simulink model "temp_control"  (Simulink 8.7)
settings: Solver=ode45  StartTime=0.0  StopTime=20000  RelTol=1e-4
settings Model: Creator=EliteBook 8470p  LastModifiedBy=EliteBook 8470p
settings DataIOCC: SignalLoggingSaveFormat=ModelDataLogs
settings OptimizationCC: BlockReduction=off  BooleanDataType=off
settings DebuggingCC: SaveWithParameterizedLinksMsg=none  SignalResolutionControl=TryResolveAllWithWarning  MultiTaskDSMMsg=warning  MultiTaskCondExecSysMsg=none
settings HardwareCC: ProdBitPerPointer=64  ProdLargestAtomicFloat=Float  ProdIntDivRoundTo=Zero  ProdEndianess=LittleEndian  ProdWordSize=64  ProdHWDeviceType=Intel->x86-64 (Windows64)  TargetUnknown=on
settings GRTTargetCC: GeneratePreprocessorConditionals=Use local settings  CombineOutputUpdateFcns=off  GRTInterface=on

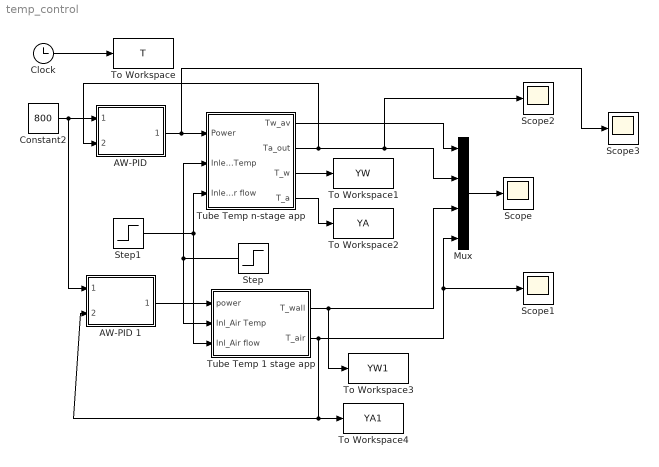
== system temp_control ==
  "AW-PID " : Subsystem  mask(Anti-windup PID){}
      mask help: Discrete PID with Anti-windup and with lowpass filter
      mask init:
      | kp=@1(1);ki=@1(2);kd=@1(3);SAM=@2;TF=@3;DT=@4;umax=@5(1);umin=@5(2);
      mask Display: disp('AW-PID+filter')
  AW-PID 1 : Subsystem  mask(Anti-windup PID){}
      mask help: Discrete PID with Anti-windup and with lowpass filter
      mask init:
      | kp=@1(1);ki=@1(2);kd=@1(3);SAM=@2;TF=@3;DT=@4;umax=@5(1);umin=@5(2);
      mask Display: disp('AW-PID+filter')
  Clock : Clock
  Constant2 : Constant  Value=800
  Mux : Mux
  Scope{,1..3} (4 alike) : Scope
  Step : Step  Time=10000  Before=25  After=500  SampleTime=0
  Step1 : Step  Time=5000  Before=1  After=10  SampleTime=0
  To Workspace : ToWorkspace  VariableName=T  SampleTime=1
  To Workspace1 : ToWorkspace  VariableName=YW  SampleTime=1
  To Workspace2 : ToWorkspace  VariableName=YA  SampleTime=1
  To Workspace3 : ToWorkspace  VariableName=YW1  SampleTime=1
  To Workspace4 : ToWorkspace  VariableName=YA1  SampleTime=1
  Tube Temp 1 stage app : Subsystem  mask{L=1, ra=.1, T_0=25, T_a0=25, T_amb=25}
      mask prompts: L "Tube length"; ra "Tube inner radius"; T_0 "Initial Tube temp"; T_a0 "Initial Air Temp"; T_amb "Ambient Temp"
      mask init:
      | cp=1078;cpa=1134;rhoa=0.5;k=2;hs=5;ha=30;
      | rhos=2500;d=.01;vt=pi*L*((ra+d)*(ra+d)-ra*ra);m=vt*rhos;
      | As=2*pi*(ra+.1)*L;V=pi*ra*ra*L;Aa=2*pi*ra*L;
      | A_d=pi*((ra+d)*(ra+d)-ra*ra);
  Tube Temp n-stage app : Subsystem  mask{L=1, n=100, ra=.1, T_01=25, T_a01=25, T_amb=25}
      mask prompts: L "Tube Length"; n "Number of sections"; ra "Tube inner radius"; T_01 "Initial tube temp"; T_a01 "Initial air temp"; T_amb "Ambient Temp"
      mask init:
      | cp=1078;cpa=1134;rhoa=0.5;hs=5;ha=30;rhos=2500;k=2;
      | d=.01;vt=pi*L*((ra+d)*(ra+d)-ra*ra);m=vt*rhos;
      | As=2*pi*(ra+.1)*L;V=pi*ra*ra*L;Aa=2*pi*ra*L;
      | A_d=pi*((ra+d)*(ra+d)-ra*ra);A_rat=1;Li=L/n;
      | T_0=T_01*ones(n,1);T_a0=T_a01*ones(n,1);
  wires:
  Mux/1 -> Scope/1
  Tube Temp 1 stage app/1(T_wall) -> Mux/3, To Workspace3/1
  Tube Temp 1 stage app/2(T_air) -> Mux/4, Scope1/1, To Workspace4/1, AW-PID 1/2(System Output)
  Tube Temp n-stage app/1(Tw_av) -> Mux/1
  Tube Temp n-stage app/2(Ta_out) -> Scope2/1, Mux/2, "AW-PID "/2(System Output)
  Clock/1 -> To Workspace/1
  Tube Temp n-stage app/3(T_w) -> To Workspace1/1
  Tube Temp n-stage app/4(T_a) -> To Workspace2/1
  Step/1 -> Tube Temp 1 stage app/2(Inl_Air Temp), Tube Temp n-stage app/2(Inlet Air Temp)
  Constant2/1 -> "AW-PID "/1(Set point), AW-PID 1/1(Set point)
  Step1/1 -> Tube Temp n-stage app/3(Inlet Air flow), Tube Temp 1 stage app/3(Inl_Air flow)
  AW-PID 1/1(Input to system) -> Tube Temp 1 stage app/1(power)
  "AW-PID "/1(Input to system) -> Scope3/1, Tube Temp n-stage app/1(Power)

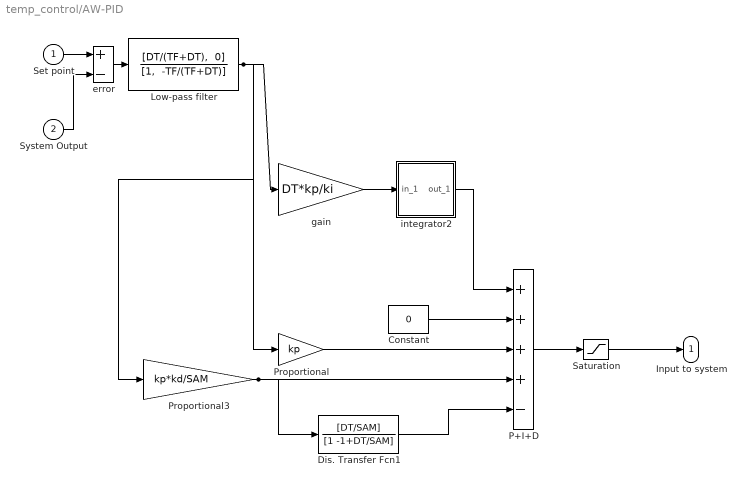
== system temp_control/AW-PID  ==
  Set point : Inport
  System Output : Inport  Port=2
  Constant : Constant  Value=0
  Dis. Transfer Fcn1 : DiscreteTransferFcn  Numerator=[DT/SAM]  Denominator=[1 -1+DT/SAM]  SampleTime=DT
  Low-pass filter : DiscreteTransferFcn  Numerator="[DT/(TF+DT),  0]"  Denominator="[1,  -TF/(TF+DT)]"  SampleTime=DT
  P+I+D : Sum  Inputs=++++-  SaturateOnIntegerOverflow=on  InputSameDT=on  OutDataTypeStr=Inherit: Same as first input
  Proportional : Gain  Gain=kp  SaturateOnIntegerOverflow=on  OutDataTypeStr=Inherit: Same as input  ParamDataTypeStr=Inherit: Same as input
  Proportional3 : Gain  Gain=kp*kd/SAM  SaturateOnIntegerOverflow=on  OutDataTypeStr=Inherit: Same as input  ParamDataTypeStr=Inherit: Same as input
  Saturation : Saturate  UpperLimit=umax  LowerLimit=umin
  error : Sum  Inputs=+-  SaturateOnIntegerOverflow=on  InputSameDT=on  OutDataTypeStr=Inherit: Same as first input
  gain : Gain  Gain=DT*kp/ki  SaturateOnIntegerOverflow=on  OutDataTypeStr=Inherit: Same as input  ParamDataTypeStr=Inherit: Same as input
  integrator2 : Subsystem  mask(Anti windup intgrator){umax=umax, umin=umin, DT=DT}
      mask prompts: DT "sampling time"
      mask help: Integral with anti-windup
      mask Display: disp('DT-I-AW')
  Input to system : Outport  InitialOutput=0
  wires:
  integrator2/1(out_1) -> P+I+D/1
  error/1 -> Low-pass filter/1
  Set point/1 -> error/1
  System Output/1 -> error/2
  Proportional3/1 -> Dis. Transfer Fcn1/1, P+I+D/4
  Low-pass filter/1 -> Proportional/1, Proportional3/1, gain/1
  Dis. Transfer Fcn1/1 -> P+I+D/5
  Proportional/1 -> P+I+D/3
  gain/1 -> integrator2/1(in_1)
  P+I+D/1 -> Saturation/1
  Saturation/1 -> Input to system/1
  Constant/1 -> P+I+D/2

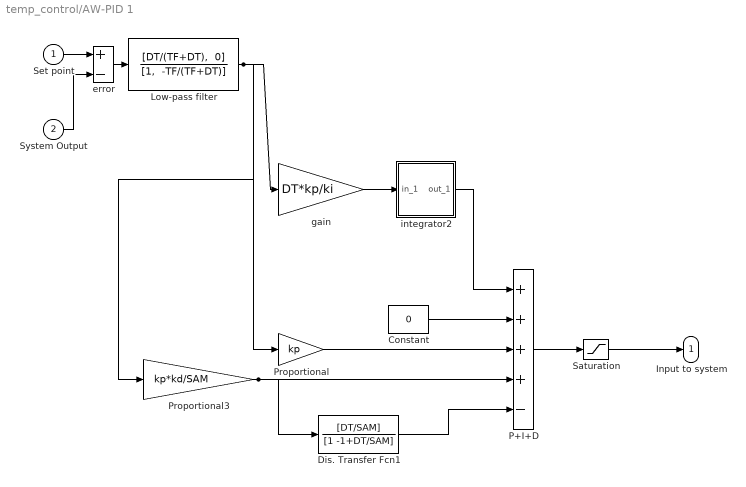
== system temp_control/AW-PID 1 ==
  Set point : Inport
  System Output : Inport  Port=2
  Constant : Constant  Value=0
  Dis. Transfer Fcn1 : DiscreteTransferFcn  Numerator=[DT/SAM]  Denominator=[1 -1+DT/SAM]  SampleTime=DT
  Low-pass filter : DiscreteTransferFcn  Numerator="[DT/(TF+DT),  0]"  Denominator="[1,  -TF/(TF+DT)]"  SampleTime=DT
  P+I+D : Sum  Inputs=++++-  SaturateOnIntegerOverflow=on  InputSameDT=on  OutDataTypeStr=Inherit: Same as first input
  Proportional : Gain  Gain=kp  SaturateOnIntegerOverflow=on  OutDataTypeStr=Inherit: Same as input  ParamDataTypeStr=Inherit: Same as input
  Proportional3 : Gain  Gain=kp*kd/SAM  SaturateOnIntegerOverflow=on  OutDataTypeStr=Inherit: Same as input  ParamDataTypeStr=Inherit: Same as input
  Saturation : Saturate  UpperLimit=umax  LowerLimit=umin
  error : Sum  Inputs=+-  SaturateOnIntegerOverflow=on  InputSameDT=on  OutDataTypeStr=Inherit: Same as first input
  gain : Gain  Gain=DT*kp/ki  SaturateOnIntegerOverflow=on  OutDataTypeStr=Inherit: Same as input  ParamDataTypeStr=Inherit: Same as input
  integrator2 : Subsystem  mask(Anti windup intgrator){umax=umax, umin=umin, DT=DT}
      mask prompts: DT "sampling time"
      mask help: Integral with anti-windup
      mask Display: disp('DT-I-AW')
  Input to system : Outport  InitialOutput=0
  wires:
  Constant/1 -> P+I+D/2
  Saturation/1 -> Input to system/1
  P+I+D/1 -> Saturation/1
  gain/1 -> integrator2/1(in_1)
  Proportional/1 -> P+I+D/3
  Dis. Transfer Fcn1/1 -> P+I+D/5
  Low-pass filter/1 -> gain/1, Proportional3/1, Proportional/1
  Proportional3/1 -> P+I+D/4, Dis. Transfer Fcn1/1
  System Output/1 -> error/2
  Set point/1 -> error/1
  error/1 -> Low-pass filter/1
  integrator2/1(out_1) -> P+I+D/1

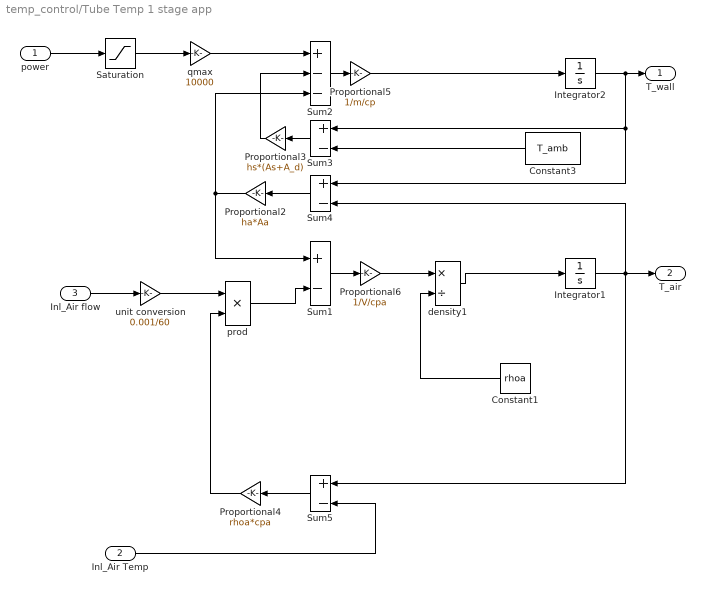
== system temp_control/Tube Temp 1 stage app ==
  power : Inport
  Inl_Air Temp : Inport  Port=2
  Inl_Air flow : Inport  Port=3
  Constant1 : Constant  Value=rhoa
  Constant3 : Constant  Value=T_amb
  Integrator1 : Integrator  InitialCondition=T_a0  UpperSaturationLimit=1  LowerSaturationLimit=0
  Integrator2 : Integrator  InitialCondition=T_0  UpperSaturationLimit=1  LowerSaturationLimit=0
  Proportional2 : Gain  Gain=ha*Aa  SaturateOnIntegerOverflow=on  OutDataTypeStr=Inherit: Same as input  ParamDataTypeStr=Inherit: Same as input
  Proportional3 : Gain  Gain=hs*(As+A_d)  SaturateOnIntegerOverflow=on  OutDataTypeStr=Inherit: Same as input  ParamDataTypeStr=Inherit: Same as input
  Proportional4 : Gain  Gain=rhoa*cpa  SaturateOnIntegerOverflow=on  OutDataTypeStr=Inherit: Same as input  ParamDataTypeStr=Inherit: Same as input
  Proportional5 : Gain  Gain=1/m/cp  SaturateOnIntegerOverflow=on  OutDataTypeStr=Inherit: Same as input  ParamDataTypeStr=Inherit: Same as input
  Proportional6 : Gain  Gain=1/V/cpa  SaturateOnIntegerOverflow=on  OutDataTypeStr=Inherit: Same as input  ParamDataTypeStr=Inherit: Same as input
  Saturation : Saturate  UpperLimit=1  LowerLimit=0
  Sum{1,3..5} (4 alike) : Sum  Inputs=+-  SaturateOnIntegerOverflow=on  InputSameDT=on  OutDataTypeStr=Inherit: Same as first input
  Sum2 : Sum  Inputs=+--  SaturateOnIntegerOverflow=on  InputSameDT=on  OutDataTypeStr=Inherit: Same as first input
  density1 : Product  Inputs=*/  SaturateOnIntegerOverflow=on  RndMeth=Zero  InputSameDT=on  OutDataTypeStr=Inherit: Same as first input
  prod : Product  Inputs=**  SaturateOnIntegerOverflow=on  RndMeth=Zero  InputSameDT=on  OutDataTypeStr=Inherit: Same as first input
  qmax : Gain  Gain=10000  SaturateOnIntegerOverflow=on  OutDataTypeStr=Inherit: Same as input  ParamDataTypeStr=Inherit: Same as input
  unit conversion : Gain  Gain=0.001/60  SaturateOnIntegerOverflow=on  OutDataTypeStr=Inherit: Same as input  ParamDataTypeStr=Inherit: Same as input
  T_wall : Outport
  T_air : Outport  Port=2
  wires:
  power/1 -> Saturation/1
  Proportional5/1 -> Integrator2/1
  Sum5/1 -> Proportional4/1
  Inl_Air Temp/1 -> Sum5/2
  Integrator1/1 -> T_air/1, Sum4/2, Sum5/1
  Sum1/1 -> Proportional6/1
  Proportional2/1 -> Sum1/1, Sum2/3
  Sum4/1 -> Proportional2/1
  Proportional3/1 -> Sum2/2
  Sum3/1 -> Proportional3/1
  Constant3/1 -> Sum3/2
  Integrator2/1 -> T_wall/1, Sum4/1, Sum3/1
  Sum2/1 -> Proportional5/1
  qmax/1 -> Sum2/1
  Constant1/1 -> density1/2
  Proportional6/1 -> density1/1
  density1/1 -> Integrator1/1
  Saturation/1 -> qmax/1
  prod/1 -> Sum1/2
  Proportional4/1 -> prod/2
  Inl_Air flow/1 -> unit conversion/1
  unit conversion/1 -> prod/1

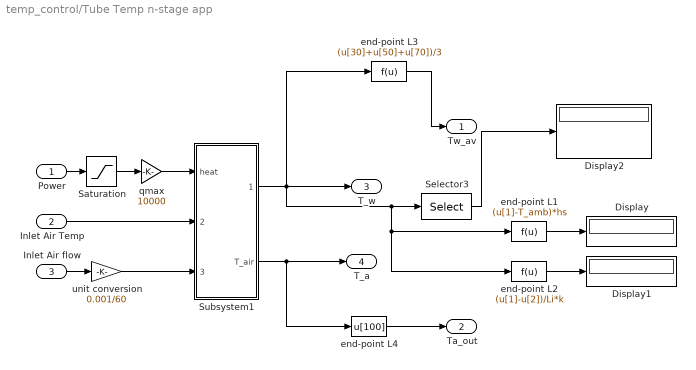
== system temp_control/Tube Temp n-stage app ==
  Power : Inport
  Inlet Air Temp : Inport  Port=2
  Inlet Air flow : Inport  Port=3
  Display : Display
      settings: Format=short_e
  Display1 : Display
      settings: Format=short_e
  Display2 : Display
      settings: Format=short_e
  Saturation : Saturate  UpperLimit=1  LowerLimit=0
  Selector3 : Selector  InputPortWidth=n  IndexOptions=Index vector (dialog)  Indices=[1,2]  OutputSizes=1
  Subsystem1 : Subsystem
  end-point L1 : Fcn  Expr=(u[1]-T_amb)*hs
  end-point L2 : Fcn  Expr=(u[1]-u[2])/Li*k
  end-point L3 : Fcn  Expr=(u[30]+u[50]+u[70])/3
  end-point L4 : Fcn  Expr=u[100]
  qmax : Gain  Gain=10000  SaturateOnIntegerOverflow=on  OutDataTypeStr=Inherit: Same as input  ParamDataTypeStr=Inherit: Same as input
  unit conversion : Gain  Gain=0.001/60  SaturateOnIntegerOverflow=on  OutDataTypeStr=Inherit: Same as input  ParamDataTypeStr=Inherit: Same as input
  Tw_av : Outport
  Ta_out : Outport  Port=2
  T_w : Outport  Port=3
  T_a : Outport  Port=4
  wires:
  end-point L2/1 -> Display1/1
  end-point L1/1 -> Display/1
  Selector3/1 -> Display2/1
  Subsystem1/2(T_air) -> end-point L4/1, T_a/1
  Subsystem1/1(T_wall) -> end-point L3/1, end-point L2/1, end-point L1/1, Selector3/1, T_w/1
  unit conversion/1 -> Subsystem1/3(Air flow)
  Inlet Air flow/1 -> unit conversion/1
  Power/1 -> Saturation/1
  Saturation/1 -> qmax/1
  Inlet Air Temp/1 -> Subsystem1/2(T_a_inlet)
  qmax/1 -> Subsystem1/1(heat)
  end-point L3/1 -> Tw_av/1
  end-point L4/1 -> Ta_out/1

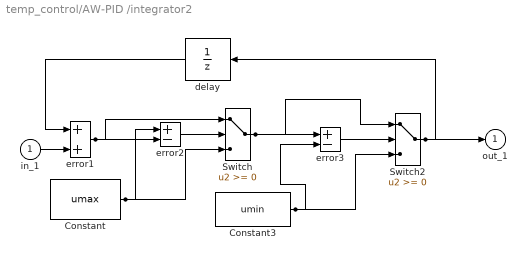
== system temp_control/AW-PID /integrator2 ==
  in_1 : Inport
  Constant : Constant  Value=umax
  Constant3 : Constant  Value=umin
  Switch : Switch  SaturateOnIntegerOverflow=on  InputSameDT=on
  Switch2 : Switch  SaturateOnIntegerOverflow=on  InputSameDT=on
  delay : DiscreteTransferFcn  Denominator=[1 0]  SampleTime=DT
  error1 : Sum  SaturateOnIntegerOverflow=on  InputSameDT=on  OutDataTypeStr=Inherit: Same as first input
  error2 : Sum  Inputs=+-  SaturateOnIntegerOverflow=on  InputSameDT=on  OutDataTypeStr=Inherit: Same as first input
  error3 : Sum  Inputs=+-  SaturateOnIntegerOverflow=on  InputSameDT=on  OutDataTypeStr=Inherit: Same as first input
  out_1 : Outport  InitialOutput=0
  wires:
  delay/1 -> error1/1
  error2/1 -> Switch/2
  Constant/1 -> error2/1, Switch/3
  error1/1 -> error2/2, Switch/1
  error3/1 -> Switch2/2
  Constant3/1 -> error3/2, Switch2/3
  Switch/1 -> error3/1, Switch2/1
  Switch2/1 -> delay/1, out_1/1
  in_1/1 -> error1/2

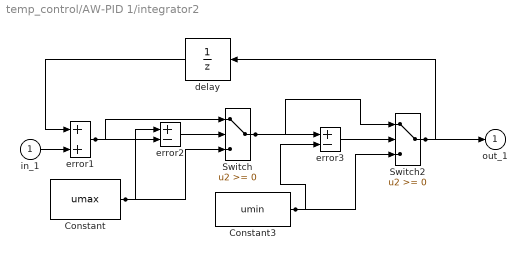
== system temp_control/AW-PID 1/integrator2 ==
  in_1 : Inport
  Constant : Constant  Value=umax
  Constant3 : Constant  Value=umin
  Switch : Switch  SaturateOnIntegerOverflow=on  InputSameDT=on
  Switch2 : Switch  SaturateOnIntegerOverflow=on  InputSameDT=on
  delay : DiscreteTransferFcn  Denominator=[1 0]  SampleTime=DT
  error1 : Sum  SaturateOnIntegerOverflow=on  InputSameDT=on  OutDataTypeStr=Inherit: Same as first input
  error2 : Sum  Inputs=+-  SaturateOnIntegerOverflow=on  InputSameDT=on  OutDataTypeStr=Inherit: Same as first input
  error3 : Sum  Inputs=+-  SaturateOnIntegerOverflow=on  InputSameDT=on  OutDataTypeStr=Inherit: Same as first input
  out_1 : Outport  InitialOutput=0
  wires:
  in_1/1 -> error1/2
  Switch2/1 -> out_1/1, delay/1
  Switch/1 -> Switch2/1, error3/1
  Constant3/1 -> Switch2/3, error3/2
  error3/1 -> Switch2/2
  error1/1 -> Switch/1, error2/2
  Constant/1 -> Switch/3, error2/1
  error2/1 -> Switch/2
  delay/1 -> error1/1

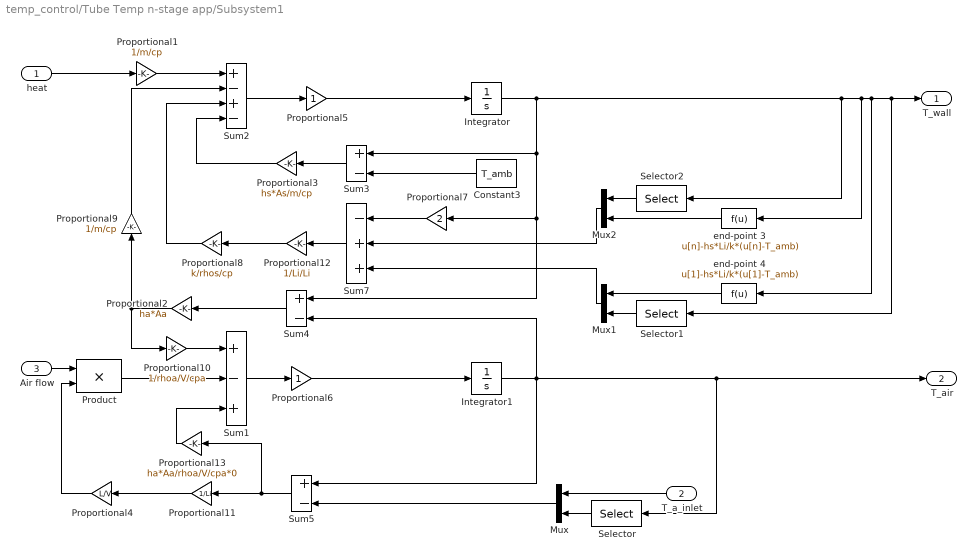
== system temp_control/Tube Temp n-stage app/Subsystem1 ==
  heat : Inport
  T_a_inlet : Inport  Port=2
  Air flow : Inport  Port=3
  Constant3 : Constant  Value=T_amb
  Integrator : Integrator  InitialCondition=T_0
  Integrator1 : Integrator  InitialCondition=T_a0
  Mux : Mux  Inputs=2
  Mux1 : Mux  Inputs=2
  Mux2 : Mux  Inputs=2
  Product : Product  SaturateOnIntegerOverflow=on  RndMeth=Zero  InputSameDT=on  OutDataTypeStr=Inherit: Same as first input
  Proportional1 : Gain  Gain=1/m/cp  SaturateOnIntegerOverflow=on  OutDataTypeStr=Inherit: Same as input  ParamDataTypeStr=Inherit: Same as input
  Proportional10 : Gain  Gain=1/rhoa/V/cpa  SaturateOnIntegerOverflow=on  OutDataTypeStr=Inherit: Same as input  ParamDataTypeStr=Inherit: Same as input
  Proportional11 : Gain  Gain=1/Li  SaturateOnIntegerOverflow=on  OutDataTypeStr=Inherit: Same as input  ParamDataTypeStr=Inherit: Same as input
  Proportional12 : Gain  Gain=1/Li/Li  SaturateOnIntegerOverflow=on  OutDataTypeStr=Inherit: Same as input  ParamDataTypeStr=Inherit: Same as input
  Proportional13 : Gain  Gain=ha*Aa/rhoa/V/cpa*0  SaturateOnIntegerOverflow=on  OutDataTypeStr=Inherit: Same as input  ParamDataTypeStr=Inherit: Same as input
  Proportional2 : Gain  Gain=ha*Aa  SaturateOnIntegerOverflow=on  OutDataTypeStr=Inherit: Same as input  ParamDataTypeStr=Inherit: Same as input
  Proportional3 : Gain  Gain=hs*As/m/cp  SaturateOnIntegerOverflow=on  OutDataTypeStr=Inherit: Same as input  ParamDataTypeStr=Inherit: Same as input
  Proportional4 : Gain  Gain=L/V  SaturateOnIntegerOverflow=on  OutDataTypeStr=Inherit: Same as input  ParamDataTypeStr=Inherit: Same as input
  Proportional5 : Gain  SaturateOnIntegerOverflow=on  OutDataTypeStr=Inherit: Same as input  ParamDataTypeStr=Inherit: Same as input
  Proportional6 : Gain  SaturateOnIntegerOverflow=on  OutDataTypeStr=Inherit: Same as input  ParamDataTypeStr=Inherit: Same as input
  Proportional7 : Gain  Gain=2  SaturateOnIntegerOverflow=on  OutDataTypeStr=Inherit: Same as input  ParamDataTypeStr=Inherit: Same as input
  Proportional8 : Gain  Gain=k/rhos/cp  SaturateOnIntegerOverflow=on  OutDataTypeStr=Inherit: Same as input  ParamDataTypeStr=Inherit: Same as input
  Proportional9 : Gain  Gain=1/m/cp  SaturateOnIntegerOverflow=on  OutDataTypeStr=Inherit: Same as input  ParamDataTypeStr=Inherit: Same as input
  Selector : Selector  InputPortWidth=n  IndexOptions=Index vector (dialog)  Indices=[1:n-1]  OutputSizes=1
  Selector1 : Selector  InputPortWidth=n  IndexOptions=Index vector (dialog)  Indices=[1:n-1]  OutputSizes=1
  Selector2 : Selector  InputPortWidth=n  IndexOptions=Index vector (dialog)  Indices=[2:n]  OutputSizes=1
  Sum1 : Sum  Inputs=+-+  SaturateOnIntegerOverflow=on  InputSameDT=on  OutDataTypeStr=Inherit: Same as first input
  Sum2 : Sum  Inputs=+-+-  SaturateOnIntegerOverflow=on  InputSameDT=on  OutDataTypeStr=Inherit: Same as first input
  Sum3 : Sum  Inputs=+-  SaturateOnIntegerOverflow=on  InputSameDT=on  OutDataTypeStr=Inherit: Same as first input
  Sum4 : Sum  Inputs=+-  SaturateOnIntegerOverflow=on  InputSameDT=on  OutDataTypeStr=Inherit: Same as first input
  Sum5 : Sum  Inputs=+-  SaturateOnIntegerOverflow=on  InputSameDT=on  OutDataTypeStr=Inherit: Same as first input
  Sum7 : Sum  Inputs=-++  SaturateOnIntegerOverflow=on  InputSameDT=on  OutDataTypeStr=Inherit: Same as first input
  end-point 3 : Fcn  Expr=u[n]-hs*Li/k*(u[n]-T_amb)
  end-point 4 : Fcn  Expr=u[1]-hs*Li/k*(u[1]-T_amb)
  T_wall : Outport
  T_air : Outport  Port=2
  wires:
  Proportional5/1 -> Integrator/1
  Proportional3/1 -> Sum2/4
  Proportional13/1 -> Sum1/3
  end-point 3/1 -> Mux2/2
  end-point 4/1 -> Mux1/1
  Selector2/1 -> Mux2/1
  Selector1/1 -> Mux1/2
  Mux/1 -> Sum5/2
  Selector/1 -> Mux/2
  T_a_inlet/1 -> Mux/1
  Air flow/1 -> Product/1
  Product/1 -> Sum1/2
  Proportional4/1 -> Product/2
  Proportional12/1 -> Proportional8/1
  Proportional11/1 -> Proportional4/1
  Proportional10/1 -> Sum1/1
  Proportional9/1 -> Sum2/2
  Proportional1/1 -> Sum2/1
  Sum2/1 -> Proportional5/1
  Integrator/1 -> end-point 3/1, end-point 4/1, Selector1/1, T_wall/1, Selector2/1, Sum3/1, Sum4/1, Proportional7/1
  Constant3/1 -> Sum3/2
  Sum3/1 -> Proportional3/1
  Sum4/1 -> Proportional2/1
  Proportional2/1 -> Proportional10/1, Proportional9/1
  Sum1/1 -> Proportional6/1
  Integrator1/1 -> T_air/1, Selector/1, Sum4/2, Sum5/1
  Sum5/1 -> Proportional13/1, Proportional11/1
  heat/1 -> Proportional1/1
  Proportional6/1 -> Integrator1/1
  Proportional7/1 -> Sum7/1
  Mux2/1 -> Sum7/2
  Mux1/1 -> Sum7/3
  Sum7/1 -> Proportional12/1
  Proportional8/1 -> Sum2/3
